simulink model "FigureBuilder"  (R2024b)
settings: Solver=VariableStepAuto  StartTime=0.0  StopTime=2  RelTol=1e-3
values from neighbouring files (symbols this model uses):
  CanaryCarrierFrequency = 20000.0    [ConfigData.sldd]
  CanaryDataRate = 100.0    [ConfigData.sldd]
  SampleRate = 48000.0    [ConfigData.sldd]
undefined symbols (not defined in the file or in its folder): DiscIntNeverNeededParam, magnitude
libraries: dspfdesign x2
settings Model: Creator=calum  LastModifiedBy=calum

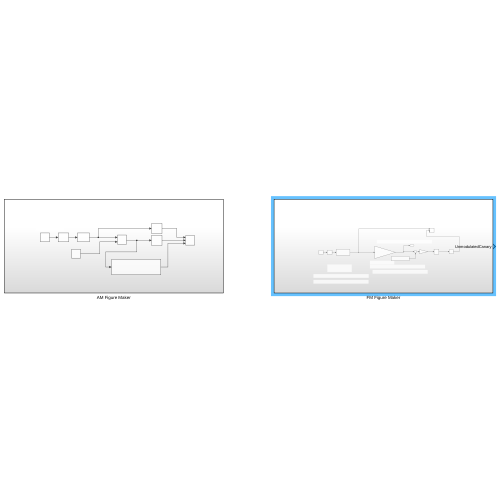
[thumbnail: Simulink's stored preview of the top-level diagram]
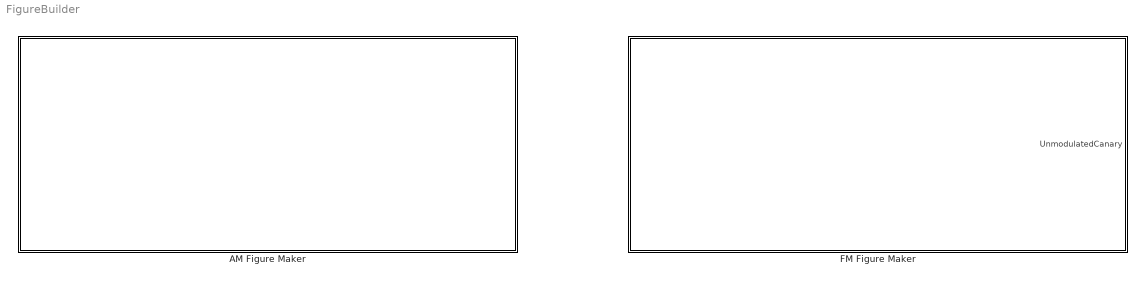
== system FigureBuilder ==
  AM Figure Maker : Subsystem
  FM Figure Maker : Subsystem

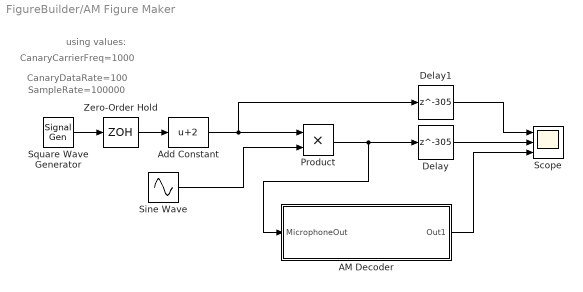
== system FigureBuilder/AM Figure Maker ==
  note: SampleRate=100000
  note: CanaryDataRate=100
  note: CanaryCarrierFreq=1000
  note: using values:
  "AM Decoder " : Subsystem  Latency=2
  Add Constant : Bias  Bias=2  SaturateOnIntegerOverflow=off
  Delay : Delay  DelayLength=305
  Delay1 : Delay  DelayLength=305
  Product : Product
  Scope : Scope  NumInputPorts=3
  Sine Wave : Sin  Frequency=CanaryCarrierFrequency*2*pi  SampleTime=1/SampleRate
  Square Wave Generator : SignalGenerator  WaveForm=square  Frequency=CanaryDataRate
  Zero-Order Hold : ZeroOrderHold  SampleTime=1/SampleRate
  wires:
  Square Wave Generator/1 -> Zero-Order Hold/1
  Sine Wave/1 -> Product/2
  Product/1 -> "AM Decoder "/1(MicrophoneOut), Delay/1
  "AM Decoder "/1(Out1) -> Scope/3
  Zero-Order Hold/1 -> Add Constant/1
  Add Constant/1 -> Delay1/1, Product/1
  Delay/1 -> Scope/2
  Delay1/1 -> Scope/1

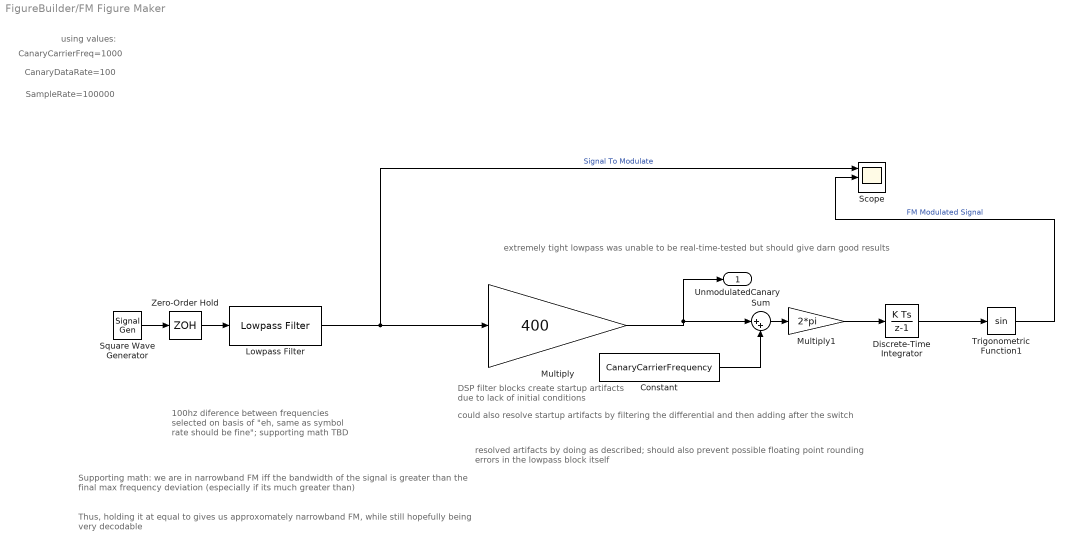
== system FigureBuilder/FM Figure Maker ==
  note: SampleRate=100000
  note: CanaryDataRate=100
  note: CanaryCarrierFreq=1000
  note: using values:
  note: DSP filter blocks create startup artifacts
      | due to lack of initial conditions
  note: Thus, holding it at equal to gives us approxomately narrowband FM, while still hopefully being very decodable
  note: extremely tight lowpass was unable to be real-time-tested but should give darn good results
  note: Supporting math: we are in narrowband FM iff the bandwidth of the signal is greater than the final max frequency deviation (especially if its much greater than)
  note: resolved artifacts by doing as described; should also prevent possible floating point rounding errors in the lowpass block itself
  note: 100hz diference between frequencies selected on basis of "eh, same as symbol rate should be fine"; supporting math TBD
  note: could also resolve startup artifacts by filtering the differential and then adding after the switch
  Constant : Constant  Value=CanaryCarrierFrequency
  Discrete-Time Integrator : DiscreteIntegrator  SampleTime=-1  ICPrevOutput=DiscIntNeverNeededParam  ICPrevScaledInput=DiscIntNeverNeededParam
  Lowpass Filter : dspfdesign/Lowpass Filter  FilterType=FIR  DesignForMinimumOrder=on  FilterOrder=50  PassbandFrequency=CanaryDataRate*2  StopbandFrequency=CanaryDataRate*6  PassbandRipple=0.1  StopbandAttenuation=80  SampleRateMode=Specify on dialog  SampleRate=SampleRate  SimulateUsing=Code generation  roundingMode=Floor  coeffsDataTypeStr=fixdt(1,16)
  Multiply : Gain  Gain=400
  Multiply1 : Gain  Gain=2*pi
  Scope : Scope  NumInputPorts=3
  Square Wave Generator : SignalGenerator  WaveForm=square  Frequency=CanaryDataRate
  Sum : Sum  Inputs=|++
  Trigonometric Function1 : Trigonometry  AngleUnit=revolution  NumberOfDataPoints=(2^16)+1
  Zero-Order Hold : ZeroOrderHold  SampleTime=1/SampleRate
  UnmodulatedCanary : Outport
  wires:
  Sum/1 -> Multiply1/1
  Trigonometric Function1/1 -> Scope/2  "FM Modulated Signal"
  Constant/1 -> Sum/2
  Discrete-Time Integrator/1 -> Trigonometric Function1/1
  Square Wave Generator/1 -> Zero-Order Hold/1
  Zero-Order Hold/1 -> Lowpass Filter/1
  Multiply1/1 -> Discrete-Time Integrator/1
  Multiply/1 -> Sum/1, UnmodulatedCanary/1
  Lowpass Filter/1 -> Scope/1, Multiply/1  "Signal To Modulate"

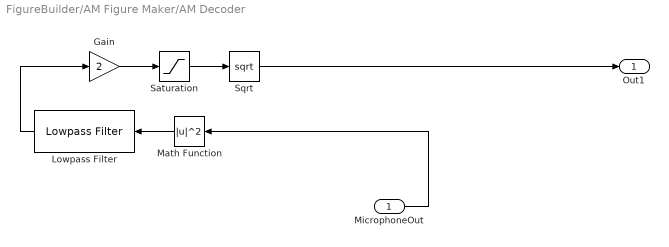
== system FigureBuilder/AM Figure Maker/AM Decoder  ==
  MicrophoneOut : Inport
  Gain : Gain  Gain=2
  Lowpass Filter : dspfdesign/Lowpass Filter  FilterType=FIR  DesignForMinimumOrder=on  FilterOrder=50  PassbandFrequency=CanaryDataRate*4  StopbandFrequency=CanaryDataRate*10  PassbandRipple=0.1  StopbandAttenuation=80  SampleRateMode=Specify on dialog  SampleRate=SampleRate  SimulateUsing=Code generation  roundingMode=Floor  coeffsDataTypeStr=fixdt(1,16)
  Math Function : Math  Operator=magnitude^2
  Saturation : Saturate  UpperLimit=inf  LowerLimit=0
  Sqrt : Sqrt
  Out1 : Outport
  wires:
  MicrophoneOut/1 -> Math Function/1
  Math Function/1 -> Lowpass Filter/1
  Saturation/1 -> Sqrt/1
  Lowpass Filter/1 -> Gain/1
  Sqrt/1 -> Out1/1
  Gain/1 -> Saturation/1
